simulink model "Massay_Sain_inv"  (R2018b)
settings: Solver=FixedStepAuto  StartTime=0.0  StopTime=1000  FixedStep=0.05  RelTol=1e-3
values from neighbouring files (symbols this model uses):
  SS_discrete = c2d(SS_full,Ts)    [discreteInverse.m]
  SS_inverse = ss(SS_inverse.A, SS_inverse.B,SS_inverse.C,SS_inverse.D,-1)    [discreteInverse.m]
undefined symbols (not defined in the file or in its folder): filterK, heave, seaWave, SS_full, surge
settings Model: Creator=user  LastModifiedBy=user

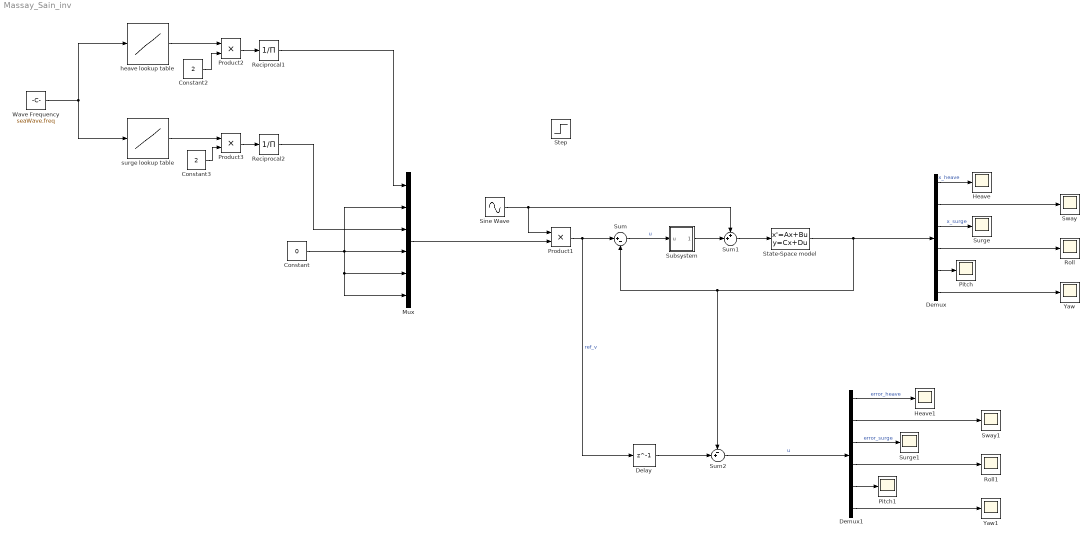
== system Massay_Sain_inv ==
  Constant : Constant  Value=0
  Constant2 : Constant  Value=2
  Constant3 : Constant  Value=2
  Delay : Delay  DelayLength=1  InitialCondition=0
  Demux : Demux  Outputs=6
  Demux1 : Demux  Outputs=6
  Heave : Scope
  Heave1 : Scope
  Mux : Mux  Inputs=6
  Pitch : Scope
  Pitch1 : Scope
  Product1 : Product
  Product2 : Product
  Product3 : Product
  Reciprocal1 : Product  Inputs=/
  Reciprocal2 : Product  Inputs=/
  Roll : Scope
  Roll1 : Scope
  Sine Wave : Sin  Amplitude=seaWave.amp  Frequency=seaWave.freq  SampleTime=0
  State-Space model : StateSpace  A=SS_full.A  B=SS_full.B  C=SS_full.C  D=SS_full.D  InitialCondition=0
  Step : Step  Time=20  SampleTime=0
  Subsystem : Subsystem
      mask Display: fprintf("K")
  Sum : Sum  Inputs=|+-
  Sum1 : Sum  Inputs=++|
  Sum2 : Sum  Inputs=-+|
  Surge : Scope
  Surge1 : Scope
  Sway : Scope
  Sway1 : Scope
  Wave Frequency : Constant  Value=seaWave.freq
  Yaw : Scope
  Yaw1 : Scope
  heave lookup table : Lookup_n-D  NumberOfTableDimensions=1  BreakpointsForDimension1=heave.freq  Table=heave.amp  InternalRulePriority=Speed  RndMeth=Simplest  InputSameDT=on
  surge lookup table : Lookup_n-D  NumberOfTableDimensions=1  BreakpointsForDimension1=surge.freq  Table=surge.amp  InternalRulePriority=Speed  RndMeth=Simplest  InputSameDT=on
  wires:
  Wave Frequency/1 -> surge lookup table/1, heave lookup table/1
  Constant/1 -> Mux/5, Mux/6, Mux/2, Mux/4
  Mux/1 -> Product1/2
  Product1/1 -> Delay/1, Sum/1  "ref_v"
  Sine Wave/1 -> Sum1/1, Product1/1
  Demux/1 -> Heave/1  "x_heave"
  Demux/3 -> Surge/1  "x_surge"
  Demux/5 -> Pitch/1
  Sum1/1 -> State-Space model/1
  Sum/1 -> Subsystem/1(u)  "u"
  Subsystem/1(Out2) -> Sum1/2
  Demux/2 -> Sway/1
  Demux/4 -> Roll/1
  Demux/6 -> Yaw/1
  heave lookup table/1 -> Product2/1
  Constant2/1 -> Product2/2
  Product2/1 -> Reciprocal1/1
  Reciprocal1/1 -> Mux/1
  surge lookup table/1 -> Product3/1
  Constant3/1 -> Product3/2
  Product3/1 -> Reciprocal2/1
  Reciprocal2/1 -> Mux/3
  Demux1/6 -> Yaw1/1
  Demux1/5 -> Pitch1/1
  Demux1/2 -> Sway1/1
  Demux1/4 -> Roll1/1
  Demux1/3 -> Surge1/1  "error_surge"
  Demux1/1 -> Heave1/1  "error_heave"
  State-Space model/1 -> Demux/1, Sum2/1, Sum/2
  Delay/1 -> Sum2/2
  Sum2/1 -> Demux1/1  "u"

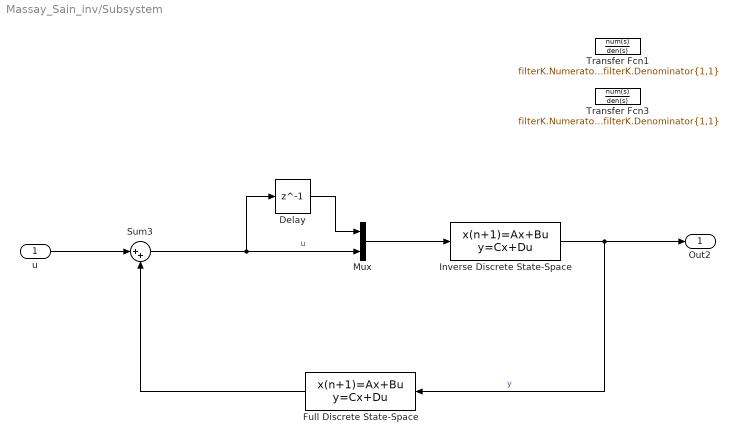
== system Massay_Sain_inv/Subsystem ==
  u : Inport
  Delay : Delay  DelayLength=1  InitialCondition=0
  Full Discrete State-Space : DiscreteStateSpace  A=SS_discrete.A  B=SS_discrete.B  C=SS_discrete.C  D=SS_discrete.D  SampleTime=-1
  Inverse Discrete State-Space : DiscreteStateSpace  A=SS_inverse.A  B=SS_inverse.B  C=SS_inverse.C  D=SS_inverse.D  SampleTime=-1
  Mux : Mux  Inputs=2
  Sum3 : Sum  Inputs=|++
  Transfer Fcn1 : TransferFcn  Numerator=filterK.Numerator{1,1}  Denominator=filterK.Denominator{1,1}
  Transfer Fcn3 : TransferFcn  Numerator=filterK.Numerator{1,1}  Denominator=filterK.Denominator{1,1}
  Out2 : Outport
  wires:
  Full Discrete State-Space/1 -> Sum3/2
  Inverse Discrete State-Space/1 -> Full Discrete State-Space/1, Out2/1  "y"
  u/1 -> Sum3/1
  Sum3/1 -> Delay/1, Mux/2  "u"
  Mux/1 -> Inverse Discrete State-Space/1
  Delay/1 -> Mux/1
